simulink model "V2_Simulink"  (R2018b)
settings: Solver=VariableStepAuto  StartTime=0.0  StopTime=20.0  RelTol=1e-3
settings Model: Creator=Asus  LastModifiedBy=Asus

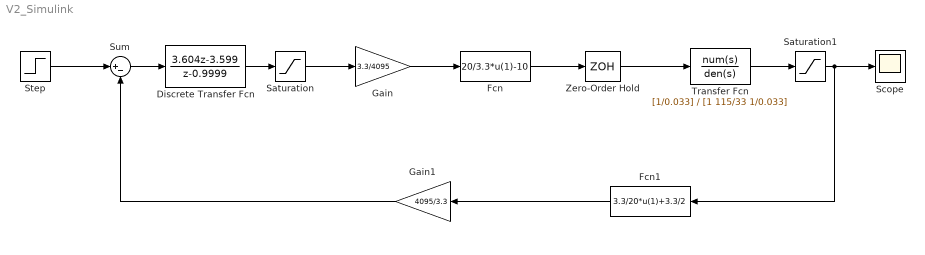
== system V2_Simulink ==
  Discrete Transfer Fcn : DiscreteTransferFcn  Numerator=[3.604 -3.599]  Denominator=[1 -0.9999]
  Fcn : Fcn  Expr=20/3.3*u(1)-10
  Fcn1 : Fcn  Expr=3.3/20*u(1)+3.3/2
  Gain : Gain  Gain=3.3/4095
  Gain1 : Gain  Gain=4095/3.3
  Saturation : Saturate  UpperLimit=4095  LowerLimit=0
  Saturation1 : Saturate  UpperLimit=10  LowerLimit=-10
  Scope : Scope
  Step : Step  Time=10  After=4095  SampleTime=0
  Sum : Sum  Inputs=|+-
  Transfer Fcn : TransferFcn  Numerator=[1/0.033]  Denominator=[1 115/33 1/0.033]
  Zero-Order Hold : ZeroOrderHold  SampleTime=0.001
  wires:
  Step/1 -> Sum/1
  Sum/1 -> Discrete Transfer Fcn/1
  Gain/1 -> Fcn/1
  Fcn/1 -> Zero-Order Hold/1
  Zero-Order Hold/1 -> Transfer Fcn/1
  Saturation/1 -> Gain/1
  Discrete Transfer Fcn/1 -> Saturation/1
  Fcn1/1 -> Gain1/1
  Gain1/1 -> Sum/2
  Saturation1/1 -> Fcn1/1, Scope/1
  Transfer Fcn/1 -> Saturation1/1
